simulink model "Albo_JL_MATLAB_No2"  (R2023b)
settings: Solver=VariableStepAuto  StartTime=0.0  StopTime=10.0  RelTol=1e-3
settings Model: Creator=ACER  LastModifiedBy=ACER

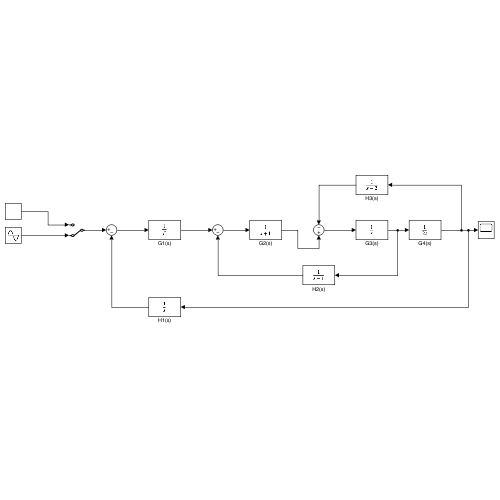
[thumbnail: Simulink's stored preview of the top-level diagram]
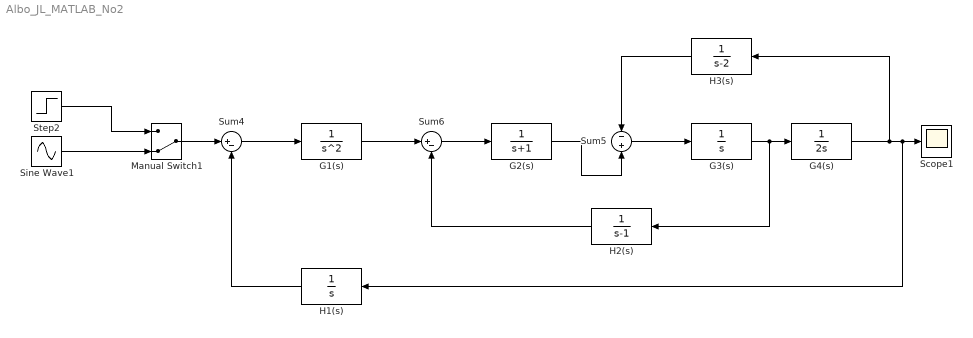
== system Albo_JL_MATLAB_No2 ==
  G1(s) : TransferFcn  Numerator=[1 ]  Denominator=[1 0 0]
  G2(s) : TransferFcn  Numerator=[1 ]  Denominator=[1 1]
  G3(s) : TransferFcn  Numerator=[1 ]  Denominator=[1 0]
  G4(s) : TransferFcn  Numerator=[1 ]  Denominator=[2 0]
  H1(s) : TransferFcn  Numerator=[1 ]  Denominator=[1 0]
  H2(s) : TransferFcn  Numerator=[1 ]  Denominator=[1 -1]
  H3(s) : TransferFcn  Denominator=[1 -2]
  Manual Switch1 : ManualSwitch  CurrentSetting=0
  Scope1 : Scope
  Sine Wave1 : Sin  SampleTime=0
  Step2 : Step  SampleTime=0
  Sum4 : Sum  Inputs=|+-
  Sum5 : Sum  Inputs=-+
  Sum6 : Sum  Inputs=|+-
  wires:
  G1(s)/1 -> Sum6/1
  G4(s)/1 -> H3(s)/1, H1(s)/1, Scope1/1
  H1(s)/1 -> Sum4/2
  H2(s)/1 -> Sum6/2
  G3(s)/1 -> H2(s)/1, G4(s)/1
  G2(s)/1 -> Sum5/2
  H3(s)/1 -> Sum5/1
  Sum6/1 -> G2(s)/1
  Sum5/1 -> G3(s)/1
  Sum4/1 -> G1(s)/1
  Step2/1 -> Manual Switch1/1
  Sine Wave1/1 -> Manual Switch1/2
  Manual Switch1/1 -> Sum4/1
